simulink model "TI_sim_with_sine"  (R2015a)
settings: Solver=ode45  StartTime=0.0  StopTime=30  RelTol=1e-3
libraries: dspsnks4 x1, dspsrcs4 x1
settings Model: Creator=ekulasek  LastModifiedBy=ekulasek

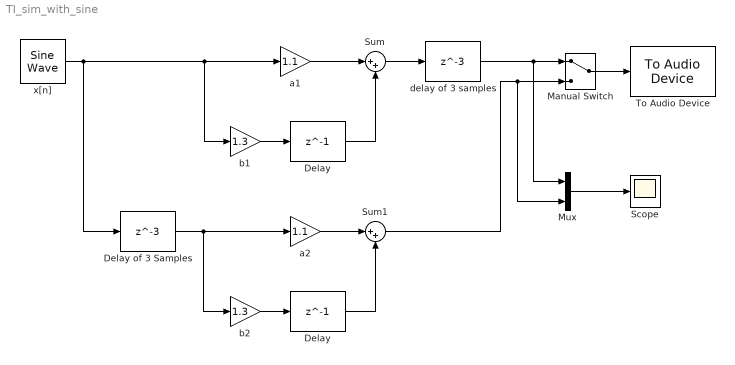
== system TI_sim_with_sine ==
  Delay : Delay  DelayLength=1  InputProcessing=Columns as channels (frame based)
  "Delay " : Delay  DelayLength=1  InputProcessing=Columns as channels (frame based)
  Delay of 3 Samples : Delay  DelayLength=3  InputProcessing=Columns as channels (frame based)
  Manual Switch : ManualSwitch
  Mux : Mux  Inputs=2
  Scope : Scope
  Sum : Sum  Inputs=|++
  Sum1 : Sum  Inputs=|++
  To Audio Device : dspsnks4/To Audio Device  deviceName=Default  inheritSampleRate=on  sampleRate=44100  deviceDatatype=Determine from input data type  autoBufferSize=on  bufferSize=4096  queueDuration=1.0  defaultOutputChannelMapping=on  outputChannelMapping=1:2  outputNumUnderrunSamples=off
  a1 : Gain  Gain=1.1
  a2 : Gain  Gain=1.1
  b1 : Gain  Gain=1.3
  b2 : Gain  Gain=1.3
  delay of 3 samples : Delay  DelayLength=3  InputProcessing=Columns as channels (frame based)
  x[n] : dspsrcs4/Sine Wave  Amplitude=1  Frequency=100  Phase=0  SampleMode=Discrete  OutComplex=Real  CompMethod=Trigonometric fcn  TableSize=Speed  SampleTime=1/1000  SamplesPerFrame=1  ResetState=Restart at time zero  dataType=double  wordLen=16  udDataType=sfix(16)  fracBitsMode=Best precision  numFracBits=15  OutDataTypeStr=double  LastOutDataTypeStr=double
  wires:
  a1/1 -> Sum/1
  b1/1 -> Delay/1
  Delay/1 -> Sum/2
  Sum/1 -> delay of 3 samples/1
  x[n]/1 -> b1/1, a1/1, Delay of 3 Samples/1
  a2/1 -> Sum1/1
  b2/1 -> "Delay "/1
  "Delay "/1 -> Sum1/2
  Delay of 3 Samples/1 -> b2/1, a2/1
  Manual Switch/1 -> To Audio Device/1
  delay of 3 samples/1 -> Manual Switch/1, Mux/1
  Sum1/1 -> Manual Switch/2, Mux/2
  Mux/1 -> Scope/1
